simulink model "gm_pemancar_bpsk"  (R2023a)
settings: Solver=FixedStepDiscrete  StartTime=0.0  StopTime=10.0  RelTol=1e-3
libraries: commrandsrc3 x1, hdlmdlgenlib x1, dspsrcs4 x1, dspsigops x1
settings Model: Creator=acer  LastModifiedBy=acer
settings SolverCC: AutoInsertRateTranBlk=on
settings OptimizationCC: BlockReduction=off  ConditionallyExecuteInputs=off  DefaultParameterBehavior=Inlined  InheritOutputTypeSmallerThanSingle=on
settings DebuggingCC: AlgebraicLoopMsg=error  InheritedTsInSrcMsg=none  SingleTaskRateTransMsg=error
settings HardwareCC: ProdBitPerPointer=32  ProdBitPerSizeT=32  ProdBitPerPtrDiffT=32  ProdLargestAtomicFloat=None  ProdIntDivRoundTo=Undefined  ProdEndianess=Unspecified  ProdWordSize=32  ProdHWDeviceType=ASIC/FPGA->ASIC/FPGA  TargetBitPerPointer=64  TargetBitPerSizeT=64  TargetBitPerPtrDiffT=64  TargetLongLongMode=on  TargetIntDivRoundTo=Zero  TargetEndianess=LittleEndian  TargetWordSize=64  TargetHWDeviceType=Custom Processor->MATLAB Host Computer  ProdEqTarget=off
settings ModelReferenceCC: EnableRefExpFcnMdlSchedulingChecks=on

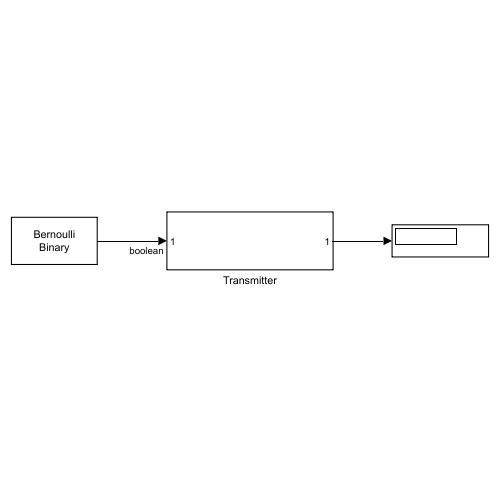
[thumbnail: Simulink's stored preview of the top-level diagram]
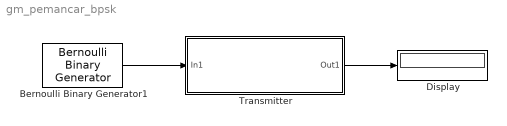
== system gm_pemancar_bpsk ==
  Bernoulli Binary Generator1 : commrandsrc3/Bernoulli Binary Generator  ProbabilityOfZero=0.5  SeedSource=Parameter  Seed=32  SampleTime=1  SamplesPerFrame=1  OutputDataType=boolean  SimulateUsing=Interpreted execution
  Display : Display
  Transmitter : Subsystem
  wires:
  Transmitter/1(Out1) -> Display/1
  Bernoulli Binary Generator1/1 -> Transmitter/1(In1)

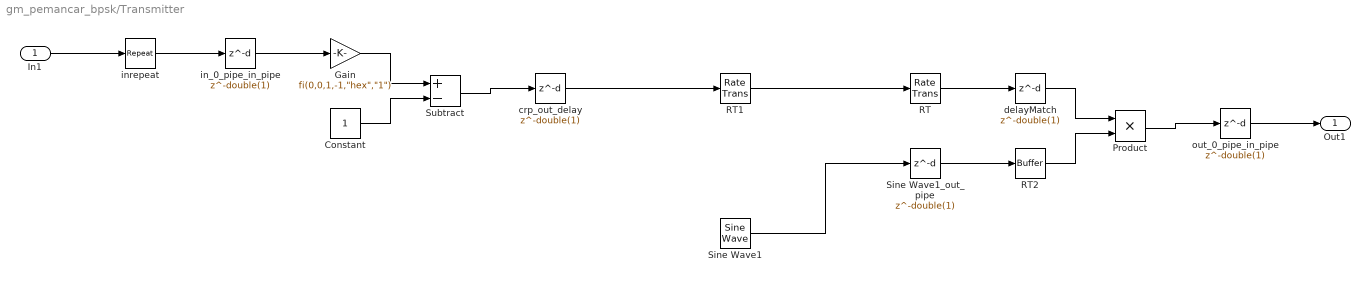
== system gm_pemancar_bpsk/Transmitter ==
  In1 : Inport  OutDataTypeStr=boolean  PortDimensions=1  SampleTime=1
  Constant : Constant  OutDataTypeStr=uint8  SampleTime=0.001
  Gain : Gain  Gain="fi(0,0,1,-1,\"hex\",\"1\")"  ParamDataTypeStr=fixdt(0, 1, -1)  OutDataTypeStr=fixdt(0, 1, -1)  SampleTime=0.001
  Product : Product  Inputs=**  OutDataTypeStr=fixdt(1, 25, 14)  SampleTime=0.001
  RT : RateTransition  Integrity=off  Deterministic=off  InitialCondition=double(0)  OutPortSampleTimeOpt=Multiple of input port sample time  OutPortSampleTimeMultiple=1/1000
  RT1 : RateTransition  OutPortSampleTimeOpt=Multiple of input port sample time  OutPortSampleTimeMultiple=1000
  RT2 : hdlmdlgenlib/Buffer
  Sine Wave1 : dspsrcs4/Sine Wave  Amplitude=1  Frequency=500  Phase=0.5*pi  SampleMode=Discrete  OutComplex=Real  CompMethod=Table lookup  TableSize=Speed  SampleTime=1/1000  SamplesPerFrame=1  ResetState=Restart at time zero  OutputFrames=off  dataType=Fixed-point  wordLen=16  udDataType=sfix(16)  fracBitsMode=Best precision  numFracBits=14  OutDataTypeStr=fixdt(1,16)  LastOutDataTypeStr=fixdt(1,16)
  Sine Wave1_out_pipe : Delay  DelayLength=double(1)  InitialCondition=0  SampleTime=0.001
  Subtract : Sum  Inputs=+-  AccumDataTypeStr=fixdt(1, 9, 0)  OutDataTypeStr=fixdt(1, 9, 0)  SampleTime=0.001
  crp_out_delay : Delay  DelayLength=double(1)  InitialCondition=0  SampleTime=0.001
  delayMatch : Delay  DelayLength=double(1)  InitialCondition=0  SampleTime=0.001
  in_0_pipe_in_pipe : Delay  DelayLength=double(1)  InitialCondition=0  SampleTime=0.001
  inrepeat : dspsigops/Repeat  FactorSource=Dialog parameter  N=double(1000)  Nmax=16  RateOptions=Allow multirate processing  ic=0  mode=Unused parameter value
  out_0_pipe_in_pipe : Delay  DelayLength=double(1)  InitialCondition=0  SampleTime=0.001
  Out1 : Outport  SampleTime=0.001
  wires:
  Sine Wave1/1 -> Sine Wave1_out_pipe/1
  In1/1 -> inrepeat/1
  delayMatch/1 -> Product/1
  Sine Wave1_out_pipe/1 -> RT2/1
  RT2/1 -> Product/2
  Product/1 -> out_0_pipe_in_pipe/1
  out_0_pipe_in_pipe/1 -> Out1/1
  inrepeat/1 -> in_0_pipe_in_pipe/1
  crp_out_delay/1 -> RT1/1
  RT1/1 -> RT/1
  RT/1 -> delayMatch/1
  Gain/1 -> Subtract/1
  Constant/1 -> Subtract/2
  Subtract/1 -> crp_out_delay/1
  in_0_pipe_in_pipe/1 -> Gain/1
